simulink model "Final_Elevator"  (R2020a)
settings: Solver=VariableStepAuto  StartTime=0.0  StopTime=inf  RelTol=1e-3
settings Model: EnablePacing=on  Creator=vivek vivian  LastModifiedBy=vivek vivian

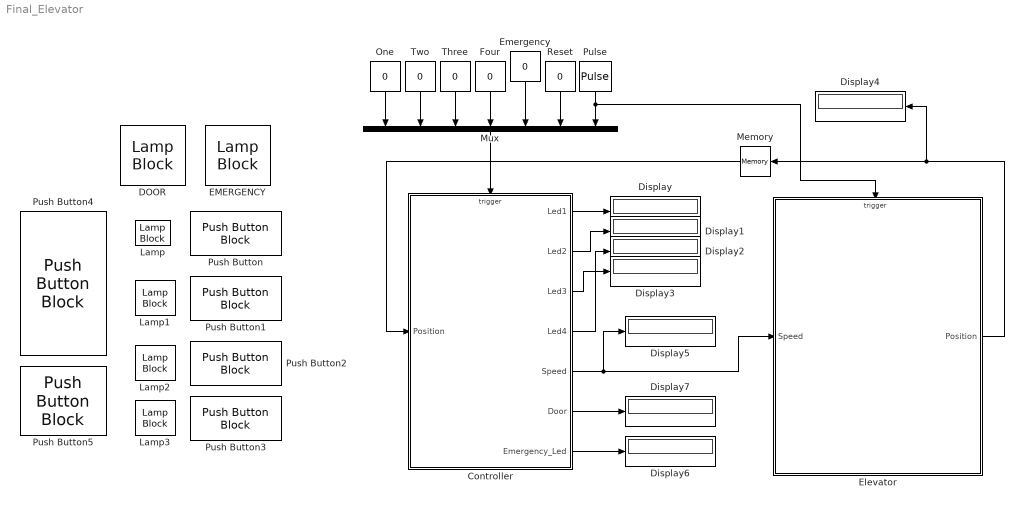
== system Final_Elevator ==
  Controller : Stateflow chart  TreatAsAtomicUnit=on
  DOOR : LampBlock
  Display{,1..7} (8 alike) : Display
  EMERGENCY : LampBlock
  Elevator : Stateflow chart  TreatAsAtomicUnit=on
  Emergency : Constant  Value=0
  Four : Constant  Value=0
  Lamp{,1..3} (4 alike) : LampBlock
  Memory : Memory  InitialCondition=1
  Mux : Mux  Inputs=7
  One : Constant  Value=0
  Pulse : DiscretePulseGenerator  PulseType=Time based  Period=10  PulseWidth=5
  Push Button : PushButtonBlock  ButtonText=One
  Push Button1 : PushButtonBlock  ButtonText=Two
  Push Button2 : PushButtonBlock  ButtonText=Three
  Push Button3 : PushButtonBlock  ButtonText=Four
  Push Button4 : PushButtonBlock  ButtonText=Emergency
  Push Button5 : PushButtonBlock  ButtonText=Reset
  Reset : Constant  Value=0
  Three : Constant  Value=0
  Two : Constant  Value=0
  wires:
  One/1 -> Mux/1
  Two/1 -> Mux/2
  Three/1 -> Mux/3
  Four/1 -> Mux/4
  Emergency/1 -> Mux/5
  Reset/1 -> Mux/6
  Mux/1 -> Controller/Trigger
  Controller/1(Led1) -> Display/1
  Controller/2(Led2) -> Display1/1
  Controller/3(Led3) -> Display2/1
  Controller/4(Led4) -> Display3/1
  Controller/5(Speed) -> Elevator/1(Speed), Display5/1
  Elevator/1(Position) -> Display4/1, Memory/1
  Memory/1 -> Controller/1(Position)
  Pulse/1 -> Elevator/Trigger, Mux/7
  Controller/6(Door) -> Display7/1
  Controller/7(Emergency_Led) -> Display6/1

== stateflow chart Final_Elevator/Elevator ==
  settings: executeAtInitialization=1
  state One
    en:Position=1;ml.lift_move(fig,Position);
  state Two
    en:Position=2;ml.lift_move(fig,Position);
  state Three
    en:Position=3;ml.lift_move(fig,Position);
  state Four
    en:Position=4;ml.lift_move(fig,Position);
  (default) -> One : {fig=ml.lift()}
  One -> Two : after(5,sec)[Speed>0]
  Two -> One [order 1] : after(5,sec)[Speed<0]
  Two -> Three [order 2] : after(5,sec)[Speed>0]
  Three -> Two [order 1] : after(5,sec)[Speed<0]
  Three -> Four [order 2] : after(5,sec)[Speed>0]
  Four -> Three : after(5,sec)[Speed<0]
  data: Speed input; Position output; fig local ml size=1
  events: TIC input RISING_EDGE_EVENT

== stateflow chart Final_Elevator/Controller ==
  settings: executeAtInitialization=1
  state Init
    en:Led1=0;Led2=0;Led3=0;Led4=0;Door=0;
  state Emergency6
    en:Emergency_Led=1;
  state First_Floor
    en:Speed=-0.2;
    on One: Led1=1;
    on Two: Led2=1;
    on Three:Led3=1;
    on Four:Led4=1;
  state Fourth_Floor
    en:Speed=0.2;
    on One: Led1=1;
    on Two: Led2=1;
    on Three:Led3=1;
    on Four:Led4=1;
  state Entry
    en:Speed=0;
    on One: Led1=1;
    on Two: Led2=1;
    on Three:Led3=1;
    on Four:Led4=1;
  state Emergency5
    en:Emergency_Led=1;
  state Emergency
    en:Emergency_Led=1;
  state Door
    en:Door=1;
    on One: Led1=1;
    on Two: Led2=1;
    on Three:Led3=1;
    on Four:Led4=1;
  state Second_Floor1
    en:Speed=0.2
    on One: Led1=1;
    on Two: Led2=1;
    on Three:Led3=1;
    on Four:Led4=1;
  state Third_Floor1_
    en:Speed=-0.2;
    on One: Led1=1;
    on Two: Led2=1;
    on Three:Led3=1;
    on Four:Led4=1;
  state Third_Floor
    en:Speed=0.2;
    on One: Led1=1;
    on Two: Led2=1;
    on Three:Led3=1;
    on Four:Led4=1;
  state Emergency3
    en:Emergency_Led=1;
  state Emergency1
    en:Emergency_Led=1;
  state Emergency4
    en:Emergency_Led=1;
  state Second_Floor
    en:Speed=-0.2;
    on One: Led1=1;
    on Two: Led2=1;
    on Three:Led3=1;
    on Four:Led4=1;
  state Emergency2
    en:Emergency_Led=1;
  (default) -> Init
  Entry -> Emergency6 [order 1] : Emergency{Speed=0;}
  Emergency6 -> Entry : Reset{Emergency_Led=0;}
  Init -> Entry
  Fourth_Floor -> Emergency5 [order 4] : Emergency{Speed=0;}
  Entry -> First_Floor [order 2] : [Led1==1]
  Entry -> Fourth_Floor [order 5] : [Led4==1]
  First_Floor -> Emergency [order 4] : Emergency{Speed=0;}
  Emergency5 -> Fourth_Floor : Reset{Emergency_Led=0;}
  Fourth_Floor -> Second_Floor1 [order 3] : [Led2==1]
  Emergency -> First_Floor : Reset{Emergency_Led=0;}
  First_Floor -> Door [order 1] : [Position==1]{Led1=0;Speed=0;}
  First_Floor -> Second_Floor [order 3] : [Led2==1]
  First_Floor -> Third_Floor1_ [order 2] : [Led3==1]
  Fourth_Floor -> Door [order 1] : [Position==4]{Led4=0;Speed=0;}
  Fourth_Floor -> Third_Floor [order 2] : [Led3==1]
  Door -> Entry : after(5,sec){Door=0;}
  Entry -> (junction 22) [order 3] : [Led2==1]
  Entry -> (junction 36) [order 4] : [Led3==1]
  Second_Floor1 -> Door [order 2] : [Position==2]{Led2=0;Speed=0;}
  Second_Floor -> Door [order 2] : [Position==2]{Led2=0;Speed=0;}
  (junction 36) -> Third_Floor1_ [order 2] : [Position>3]
  (junction 22) -> Second_Floor1 [order 1] : [Position<2]
  (junction 36) -> Third_Floor [order 1] : [Position<3]
  (junction 22) -> Second_Floor [order 2] : [Position>2]
  Third_Floor1_ -> Door [order 2] : [Position==3]{Led3=0;Speed=0;}
  Third_Floor -> Door [order 2] : [Position==3]{Led3=0;Speed=0;}
  Second_Floor1 -> Emergency1 [order 1] : Emergency{Speed=0;}
  Third_Floor -> Emergency3 [order 1] : Emergency{Speed=0;}
  Emergency4 -> Third_Floor1_ : Reset{Emergency_Led=0;}
  Emergency1 -> Second_Floor1 : Reset{Emergency_Led=0;}
  Third_Floor -> Second_Floor1 [order 3] : [Led2==1]
  Second_Floor -> Third_Floor1_ [order 3] : [Led3==1]
  Third_Floor1_ -> Emergency4 [order 1] : Emergency{Speed=0;}
  Emergency3 -> Third_Floor : Reset{Emergency_Led=0;}
  Second_Floor -> Emergency2 [order 1] : Emergency{Speed=0;}
  Emergency2 -> Second_Floor : Reset{Emergency_Led=0;}
  data: Led1 output double; Led2 output double; Led3 output double; Led4 output double; Speed output double; Position input double; Door output double; Emergency_Led output double
  events: One input RISING_EDGE_EVENT; Two input RISING_EDGE_EVENT; Three input RISING_EDGE_EVENT; Four input RISING_EDGE_EVENT; Emergency input RISING_EDGE_EVENT; Reset input RISING_EDGE_EVENT; TIC input RISING_EDGE_EVENT
